simulink model "MPSLab2"  (R2014b)
settings: Solver=ode45  StartTime=0.0  StopTime=30  RelTol=1e-3
undefined symbols (not defined in the file): sigbuilder_block
settings Model: Creator=kiril_000  LastModifiedBy=kiril_000

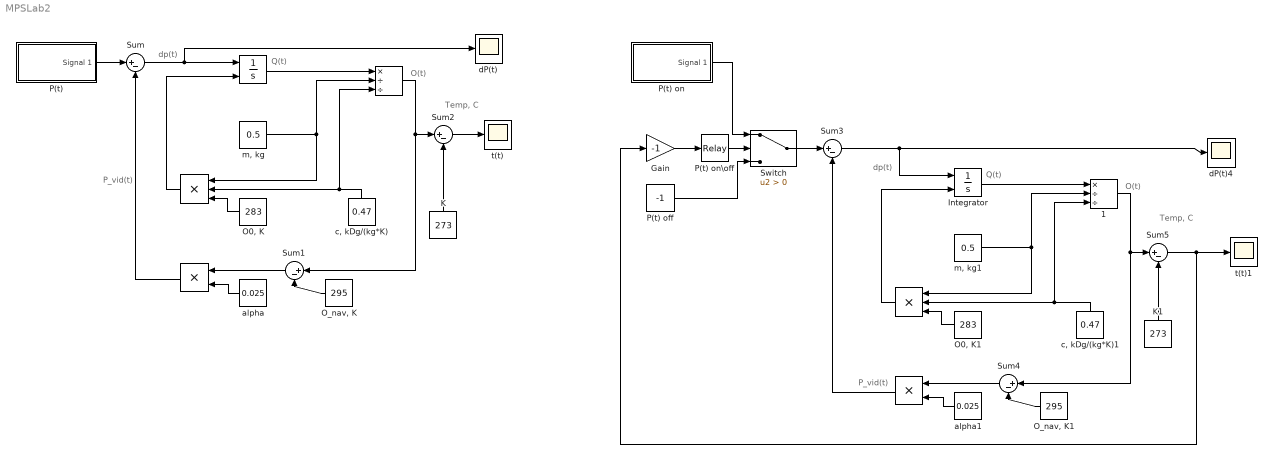
== system MPSLab2 ==
  note: O(t)
  note: Temp, C
  note: P_vid(t)
  note: Q(t)
  note: dp(t)
  note: O(t)
  note: Temp, C
  note: P_vid(t)
  note: Q(t)
  note: dp(t)
  " " : Product  Inputs=3
  "  " : Product
  "   " : Integrator  InitialConditionSource=external
  "    " : Product  Inputs=*//
  "          " : Product  Inputs=3
  "                    " : Product
  "    1" : Product  Inputs=*//
  "   Integrator" : Integrator  InitialConditionSource=external
  Gain : Gain  Gain=-1
  K : Constant  Value=273
  K1 : Constant  Value=273
  "O0, K" : Constant  Value=283
  "O0, K1" : Constant  Value=283
  "O_nav, K" : Constant  Value=295
  "O_nav, K1" : Constant  Value=295
  P(t) : Subsystem  Tag=STV Subsys  LoadFcn=sigbuilder_block('load');  StartFcn=sigbuilder_block('start');  StopFcn=sigbuilder_block('stop');  ClipboardFcn=sigbuilder_block('clipboard');  mask(Sigbuilder block){}
      mask help: Simulink:masks:SigbuilderBlock_MD
      mask init:
      | if ~strcmp(get_param(bdroot(gcbh),'SimulationStatus'),'stopped') tuvar = sigbuilder_block('maskInit'); end
      settings: CopyFcn=sigbuilder_block('copy');  DeleteFcn=sigbuilder_block('delete');  ModelCloseFcn=sigbuilder_block('modelClose');  PreSaveFcn=sigbuilder_block('preSave');  PauseFcn=sigbuilder_block('pause');  ContinueFcn=sigbuilder_block('continue');  NameChangeFcn=sigbuilder_block('namechange');  OpenFcn=sigbuilder_block('open',[437.6 199.2 550.4 400 ]);  CloseFcn=sigbuilder_block('close');
      mask Display: plot(0, 0, 100, 100,[2, 2, 32, 32, 2], [68, 8, 8, 68, 68],[32, 2], [38, 38], [32, 19, 2],[53, 60, 44], [32, 17, 17, 2],[16, 16, 31, 31]);txt = getActiveGroup(gcbh);text(2, 100, txt,'verticalAlignment', 'top');
  P(t) off : Constant  Value=-1
  P(t) on : Subsystem  Tag=STV Subsys  LoadFcn=sigbuilder_block('load');  StartFcn=sigbuilder_block('start');  StopFcn=sigbuilder_block('stop');  ClipboardFcn=sigbuilder_block('clipboard');  mask(Sigbuilder block){}
      mask help: Simulink:masks:SigbuilderBlock_MD
      mask init:
      | if ~strcmp(get_param(bdroot(gcbh),'SimulationStatus'),'stopped') tuvar = sigbuilder_block('maskInit'); end
      settings: CopyFcn=sigbuilder_block('copy');  DeleteFcn=sigbuilder_block('delete');  ModelCloseFcn=sigbuilder_block('modelClose');  PreSaveFcn=sigbuilder_block('preSave');  PauseFcn=sigbuilder_block('pause');  ContinueFcn=sigbuilder_block('continue');  NameChangeFcn=sigbuilder_block('namechange');  OpenFcn=sigbuilder_block('open',[437.6 199.2 550.4 400 ]);  CloseFcn=sigbuilder_block('close');
      mask Display: plot(0, 0, 100, 100,[2, 2, 32, 32, 2], [68, 8, 8, 68, 68],[32, 2], [38, 38], [32, 19, 2],[53, 60, 44], [32, 17, 17, 2],[16, 16, 31, 31]);txt = getActiveGroup(gcbh);text(2, 100, txt,'verticalAlignment', 'top');
  P(t) on\off : Relay  OnSwitchValue=-15  OffSwitchValue=-28
  Sum{,1..5} (6 alike) : Sum  Inputs=|+-
  Switch : Switch  Criteria=u2 > Threshold
  alpha : Constant  Value=0.025
  alpha1 : Constant  Value=0.025
  "c, kDg/(kg*K)" : Constant  Value=0.47
  "c, kDg/(kg*K)1" : Constant  Value=0.47
  dP(t) : Scope
      settings: TimeRange=30  YMin=0.1  YMax=0.7000000000000001  SaveName=ScopeData2
  dP(t)4 : Scope
      settings: TimeRange=30  YMin=0.118  YMax=0.136  SaveName=ScopeData8
  "m, kg" : Constant  Value=0.5
  "m, kg1" : Constant  Value=0.5
  t(t) : Scope
  t(t)1 : Scope
      settings: YMin=8.2  YMax=10  SaveName=ScopeData3
  wires:
  "O0, K"/1 -> " "/3
  "c, kDg/(kg*K)"/1 -> " "/2, "    "/3
  "m, kg"/1 -> "    "/2, " "/1
  "   "/1 -> "    "/1
  alpha/1 -> "  "/2
  Sum1/1 -> "  "/1
  "O_nav, K"/1 -> Sum1/2
  K/1 -> Sum2/2
  "    "/1 -> Sum2/1, Sum1/1
  Sum2/1 -> t(t)/1
  Sum/1 -> dP(t)/1, "   "/1
  " "/1 -> "   "/2
  "  "/1 -> Sum/2
  P(t)/1(Signal 1) -> Sum/1
  "O0, K1"/1 -> "          "/3
  "c, kDg/(kg*K)1"/1 -> "    1"/3, "          "/2
  "m, kg1"/1 -> "          "/1, "    1"/2
  "   Integrator"/1 -> "    1"/1
  alpha1/1 -> "                    "/2
  Sum4/1 -> "                    "/1
  "O_nav, K1"/1 -> Sum4/2
  K1/1 -> Sum5/2
  "    1"/1 -> Sum4/1, Sum5/1
  Sum5/1 -> Gain/1, t(t)1/1
  Sum3/1 -> "   Integrator"/1, dP(t)4/1
  "          "/1 -> "   Integrator"/2
  "                    "/1 -> Sum3/2
  P(t) on/1(Signal 1) -> Switch/1
  Switch/1 -> Sum3/1
  P(t) on\off/1 -> Switch/2
  Gain/1 -> P(t) on\off/1
  P(t) off/1 -> Switch/3

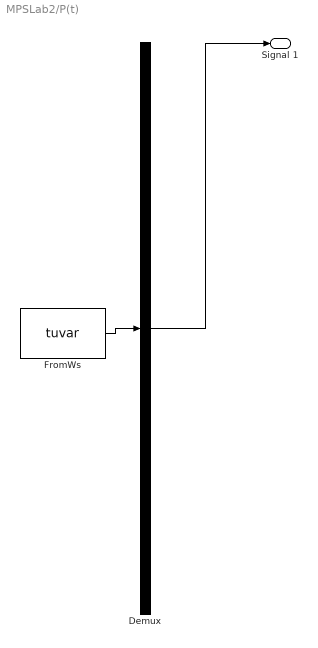
== system MPSLab2/P(t) ==
  Demux : Demux  Tag=STV Demux  Outputs=1
  FromWs : FromWorkspace  Tag=STV FromWs  VariableName=tuvar  SampleTime=0
      SigBuilderData=|
      | common.afterFinalStr = 'Extrapolate'
      | common.sampleTime = 0
      | dataSet.timeRange = [0 20]
      | dataSet.name = 'Group 1'
      | sbobj.Groups.Name = 'Group 1'
      | sbobj.Groups.Signals.Name = 'Signal 1'
      | sbobj.Groups.Signals.XData = [0 2 12 20]
      | sbobj.Groups.Signals.YData = [0 0 1 1]
      | sbobj.Groups.TimeRange = [0 20]
  Signal 1 : Outport  Tag=STV Outport
  wires:
  Demux/1 -> Signal 1/1
  FromWs/1 -> Demux/1

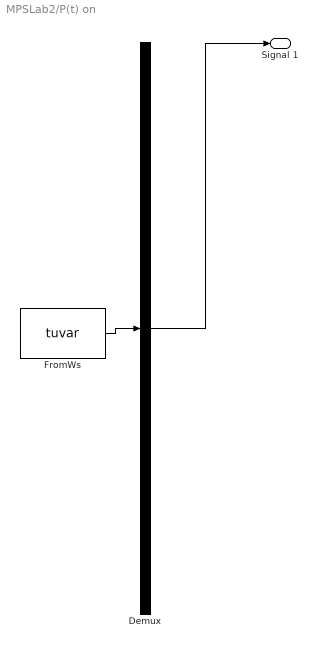
== system MPSLab2/P(t) on ==
  Demux : Demux  Tag=STV Demux  Outputs=1
  FromWs : FromWorkspace  Tag=STV FromWs  VariableName=tuvar  SampleTime=0
      SigBuilderData=|
      | common.afterFinalStr = 'Extrapolate'
      | common.sampleTime = 0
      | dataSet.timeRange = [0 20]
      | dataSet.name = 'Group 1'
      | sbobj.Groups.Name = 'Group 1'
      | sbobj.Groups.Signals.Name = 'Signal 1'
      | sbobj.Groups.Signals.XData = [0 2 12 20]
      | sbobj.Groups.Signals.YData = [0 0 1 1]
      | sbobj.Groups.TimeRange = [0 20]
  Signal 1 : Outport  Tag=STV Outport
  wires:
  FromWs/1 -> Demux/1
  Demux/1 -> Signal 1/1
